simulink model "liti1"  (Simulink 5.0)
settings: Solver=ode4  SolverMode=SingleTasking  StartTime=0.0  StopTime=10  FixedStep=0.001  RelTol=1e-3
libraries: cstblocks x1
settings Model: LastModifiedBy=Administrator

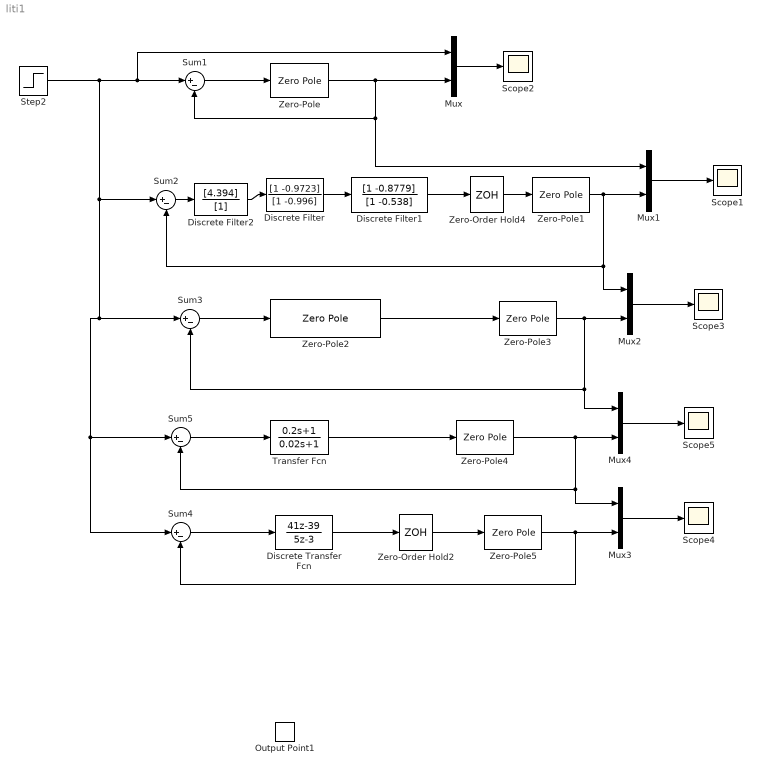
== system liti1 ==
  Discrete Transfer Fcn : DiscreteTransferFcn  Numerator=[41 -39]  Denominator=[5 -3]  SampleTime=0.01
  Discrete Filter : DiscreteFilter  Numerator=[1 -0.9723]  Denominator=[1 -0.996]  SampleTime=0.1
  Discrete Filter1 : DiscreteFilter  Numerator=[1 -0.8779]  Denominator=[1 -0.538]  SampleTime=0.1
  Discrete Filter2 : DiscreteFilter  Numerator=[4.394]  Denominator=[1]  SampleTime=0.1
  Mux{,1..4} (5 alike) : Mux  Inputs=2
  Output Point1 : cstblocks/Output Point
  Scope{1..5} (5 alike) : Scope
      Scope1 settings: YMin=-3.5  YMax=1  MaxDataPoints=500000
      Scope2 settings: YMin=-3.5  YMax=1  MaxDataPoints=500000
      Scope3 settings: YMin=-3.5  YMax=1  SaveName=ScopeData2  MaxDataPoints=500000
      Scope4 settings: YMin=-3.5  YMax=1  SaveName=ScopeData3  MaxDataPoints=500000
      Scope5 settings: YMin=-3.5  YMax=1  SaveName=ScopeData4  MaxDataPoints=500000
  Step2 : Step  Time=0  SampleTime=0
  Sum{1..5} (5 alike) : Sum  Inputs=|+-  SaturateOnIntegerOverflow=on
  Transfer Fcn : TransferFcn  Numerator=[0.2 1]  Denominator=[0.02 1]
  Zero-Order Hold2 : ZeroOrderHold  SampleTime=0.01
  Zero-Order Hold4 : ZeroOrderHold  SampleTime=0.1
  Zero-Pole{,1,3..4} (4 alike) : ZeroPole  Zeros=[]  Poles=[0 -2]  Gain=[4]
  Zero-Pole2 : ZeroPole  Zeros=[-0.28 -1.3]  Poles=[-0.04 -6]  Gain=[5.3]
  Zero-Pole5 : ZeroPole  Zeros=[]  Poles=[0 -2]  Gain=[12]
  wires:
  Sum1/1 -> Zero-Pole/1
  Mux/1 -> Scope2/1
  Zero-Pole/1 -> Mux/2, Sum1/2, Mux1/1
  Step2/1 -> Mux/1, Sum1/1, Sum2/1, Sum3/1, Sum5/1, Sum4/1
  Sum2/1 -> Discrete Filter2/1
  Mux1/1 -> Scope1/1
  Zero-Pole1/1 -> Mux1/2, Sum2/2, Mux2/1
  Discrete Filter1/1 -> Zero-Order Hold4/1
  Zero-Order Hold4/1 -> Zero-Pole1/1
  Discrete Filter/1 -> Discrete Filter1/1
  Discrete Filter2/1 -> Discrete Filter/1
  Mux2/1 -> Scope3/1
  Zero-Pole3/1 -> Mux2/2, Sum3/2, Mux4/1
  Zero-Pole2/1 -> Zero-Pole3/1
  Sum3/1 -> Zero-Pole2/1
  Mux3/1 -> Scope4/1
  Zero-Pole5/1 -> Mux3/2, Sum4/2
  Zero-Order Hold2/1 -> Zero-Pole5/1
  Discrete Transfer Fcn/1 -> Zero-Order Hold2/1
  Sum4/1 -> Discrete Transfer Fcn/1
  Mux4/1 -> Scope5/1
  Zero-Pole4/1 -> Mux4/2, Sum5/2, Mux3/1
  Transfer Fcn/1 -> Zero-Pole4/1
  Sum5/1 -> Transfer Fcn/1
